simulink model "DP2_Jason_Li"  (R2022a)
settings: Solver=VariableStepAuto  StartTime=0.0  StopTime=100  RelTol=1e-3
model workspace (MATLAB code in the model file):
  | current1=110;
  | current2=110;
  | current3=0;
  | current4=200;
  | const_v=675;
  | 
  | v_set_1=current1*0.3;
  | 
  | v_set_2=current2*0.3;
  | 
  | v_set_3=current3*0.3;
  | 
  | v_set_4=current4*0.3;
  | 
  | P=12;
  | I=1;
  | D=12;
undefined symbols (not defined in the file): D11, Delta, Ion, Lithium
libraries: spsDiodeLib x32, spsSeriesRLCBranchLib x22, spsCurrentMeasurementLib x16, simulink x12, spsMosfetLib x8, slpidlib x8, spsTriangleGeneratorLib x8, spsBatteryLib x4, spsVariableResistorLib x4, spsVoltageMeasurementLib x4, spsThreePhaseTransformerThreeWindingsLib x1, spsThreePhaseVIMeasurementLib x1
(part 2 of 2)

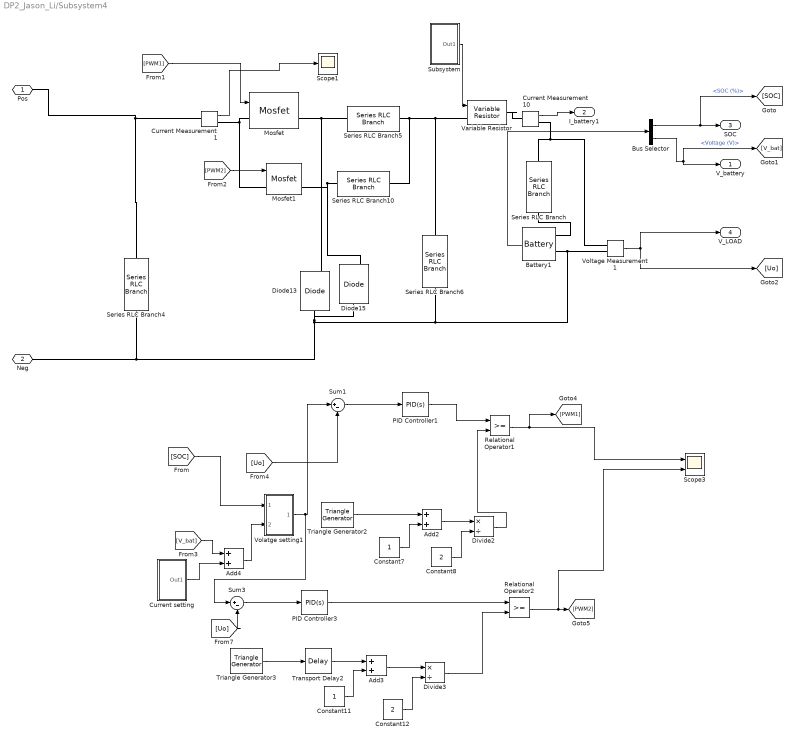
== system DP2_Jason_Li/Subsystem4 ==
  Add2 : Sum
  Add3 : Sum
  Add4 : Sum
  Battery1 : spsBatteryLib/Battery  BatType=Lithium-Ion  ShowTempParam=off  ThermalPreset=no  ShowAgeParam=off  NomV=600  NomQ=150  SOC=0  Batt_Tr=1  PresetModel=off  MaxQ=150  MinV=450  FullV=660  Dis_rate=65.2174  R=1e-7  Normal_OP=135.6522  expZone="[648.2315      7.369565]"  current=[6.5 13 32.5]  Units=Time  Tci=20  NomT=20  T2=-30  MaxQ2=4.8  FullV2=7.1  Normal_OP2=5.655  expZone2="[6.58           1]"  Rca=0.6  ti=2000  Dp=0  Neq0=0  Tsim=1e6  Ta1=25  Qeol=5.4*0.9  Reol=0.013333*1.2  Char_age=[2.3478, 3]  Dis_age=[2.3478, 10]  N1=1500  N2=10500  N3=1000  N4=1400  Ta2=45  N5=950
  Bus Selector : BusSelector  OutputSignals=SOC (%),Voltage (V)
  Constant11 : Constant
  Constant12 : Constant  Value=2
  Constant7 : Constant
  Constant8 : Constant  Value=2
  Current Measurement1 : spsCurrentMeasurementLib/Current Measurement  PhasorSimulation=off  OutputType=Complex  PSBequivalent=0
  Current Measurement10 : spsCurrentMeasurementLib/Current Measurement  PhasorSimulation=off  OutputType=Complex  PSBequivalent=0
  Current setting : Subsystem
  Diode13 : spsDiodeLib/Diode  Ron=0.0001  Lon=0  Vf=0.0001  IC=0  UseSnubber=0  Rs=500  Cs=250e-9  Measurements=on
  Diode15 : spsDiodeLib/Diode  Ron=0.0001  Lon=0  Vf=0.0001  IC=0  UseSnubber=0  Rs=500  Cs=250e-9  Measurements=on
  Divide2 : Product  Inputs=*/
  Divide3 : Product  Inputs=*/
  Mosfet : spsMosfetLib/Mosfet  Ron=0.1  Lon=0  Rd=0.01  Vfd=0  IC=0  Rs=1e5  Cs=inf  Measurements=on
  Mosfet1 : spsMosfetLib/Mosfet  Ron=0.1  Lon=0  Rd=0.01  Vfd=0  IC=0  Rs=1e5  Cs=inf  Measurements=on
  PID Controller1 : slpidlib/PID Controller  Controller=PID  Form=Parallel  TimeDomain=Continuous-time  UseExternalTs=off  SampleTime=-1  IntegratorMethod=Forward Euler  FilterMethod=Forward Euler  ControllerParametersSource=internal  P=P  I=I  UseKiTs=off  D=D  N=100  UseFilter=on  TunerSelectOption=Frequency Response Based  InitialConditionSource=internal  InitialConditionForIntegrator=0  InitialConditionForFilter=0  DifferentiatorICPrevScaledInput=0  ExternalReset=none  TrackingMode=off  Kt=1  LimitOutput=off  SatLimitsSource=internal  UpperSaturationLimit=inf  LowerSaturationLimit=-inf  LinearizeAsGain=on  AntiWindupMode=none  Kb=1  POutMin=[]  POutMax=[]  IOutMin=[]  IOutMax=[]  DOutMin=[]  DOutMax=[]  NOutMin=[]  NOutMax=[]  SumOutMin=[]  SumOutMax=[]  SaturationOutMin=[]  SaturationOutMax=[]  PParamMin=[]  PParamMax=[]  IParamMin=[]  IParamMax=[]  DParamMin=[]  DParamMax=[]  NParamMin=[]  NParamMax=[]  KbParamMin=[]  KbParamMax=[]  KtParamMin=[]  KtParamMax=[]  KbOutMin=[]  KbOutMax=[]  KtOutMin=[]  KtOutMax=[]  IntegratorOutMin=[]  IntegratorOutMax=[]  FilterOutMin=[]  FilterOutMax=[]  SumI1OutMin=[]  SumI1OutMax=[]  SumI2OutMin=[]  SumI2OutMax=[]  SumI3OutMin=[]  SumI3OutMax=[]  SumI4OutMin=[]  SumI4OutMax=[]  SumDOutMin=[]  SumDOutMax=[]  DifferentiatorOutMin=[]  DifferentiatorOutMax=[]  FilterDiffOutCoefMin=[]  FilterDiffOutCoefMax=[]  ReciprocalOutMin=[]  ReciprocalOutMax=[]  SumDenOutMin=[]  SumDenOutMax=[]  SumNumOutMin=[]  SumNumOutMax=[]  DivideOutMin=[]  DivideOutMax=[]  UdiffTsProdOutMin=[]  UdiffTsProdOutMax=[]  NTsProdOutMin=[]  NTsProdOutMax=[]  UintegralTsProdOutMin=[]  UintegralTsProdOutMax=[]  UngainTsProdOutMin=[]  UngainTsProdOutMax=[]  IntegratorContinuousStateAttributes=''  IntegratorStateMustResolveToSignalObject=off  IntegratorRTWStateStorageClass=Auto  FilterContinuousStateAttributes=''  FilterStateMustResolveToSignalObject=off  FilterRTWStateStorageClass=Auto  ParallelPVariant=InternalParameters  IdealPVariant=Disabled  IVariant=InternalParameters  DVariant=InternalParameters  IntegratorVariant=Continuous  SatVariant=Disabled  AWVariant=Passthrough  PCopyVariant=Disabled  TRVariant=Disabled  FdbkBlocksVariant=Forward  IdealPFdbkVariant=Disabled  SatFdbkVariant=Disabled  DerivativeFilterVariant=ContFilter  NVariant=InternalParameters  NCopyVariant=Disabled  FilterICVariant=InternalICsFilter  IntegratorICVariant=InternalICs  ExternalResetVariant=Disabled  TRSumVariant=Passthrough  SumFdbkVariant=Disabled  SumVariant=Sum_PID  TsampFilterVariant=InternalTs  TsampNgainVariant=Passthrough  TsampIntegralVariant=Passthrough  ExternalSaturationOutDataTypeStr=Inherit: Same as second input  aMode=0
  PID Controller3 : slpidlib/PID Controller  Controller=PID  Form=Parallel  TimeDomain=Continuous-time  UseExternalTs=off  SampleTime=-1  IntegratorMethod=Forward Euler  FilterMethod=Forward Euler  ControllerParametersSource=internal  P=P  I=I  UseKiTs=off  D=D  N=100  UseFilter=on  TunerSelectOption=Transfer Function Based (PID Tuner App)  InitialConditionSource=internal  InitialConditionForIntegrator=0  InitialConditionForFilter=0  DifferentiatorICPrevScaledInput=0  ExternalReset=none  TrackingMode=off  Kt=1  LimitOutput=off  SatLimitsSource=internal  UpperSaturationLimit=inf  LowerSaturationLimit=-inf  LinearizeAsGain=on  AntiWindupMode=none  Kb=1  POutMin=[]  POutMax=[]  IOutMin=[]  IOutMax=[]  DOutMin=[]  DOutMax=[]  NOutMin=[]  NOutMax=[]  SumOutMin=[]  SumOutMax=[]  SaturationOutMin=[]  SaturationOutMax=[]  PParamMin=[]  PParamMax=[]  IParamMin=[]  IParamMax=[]  DParamMin=[]  DParamMax=[]  NParamMin=[]  NParamMax=[]  KbParamMin=[]  KbParamMax=[]  KtParamMin=[]  KtParamMax=[]  KbOutMin=[]  KbOutMax=[]  KtOutMin=[]  KtOutMax=[]  IntegratorOutMin=[]  IntegratorOutMax=[]  FilterOutMin=[]  FilterOutMax=[]  SumI1OutMin=[]  SumI1OutMax=[]  SumI2OutMin=[]  SumI2OutMax=[]  SumI3OutMin=[]  SumI3OutMax=[]  SumI4OutMin=[]  SumI4OutMax=[]  SumDOutMin=[]  SumDOutMax=[]  DifferentiatorOutMin=[]  DifferentiatorOutMax=[]  FilterDiffOutCoefMin=[]  FilterDiffOutCoefMax=[]  ReciprocalOutMin=[]  ReciprocalOutMax=[]  SumDenOutMin=[]  SumDenOutMax=[]  SumNumOutMin=[]  SumNumOutMax=[]  DivideOutMin=[]  DivideOutMax=[]  UdiffTsProdOutMin=[]  UdiffTsProdOutMax=[]  NTsProdOutMin=[]  NTsProdOutMax=[]  UintegralTsProdOutMin=[]  UintegralTsProdOutMax=[]  UngainTsProdOutMin=[]  UngainTsProdOutMax=[]  IntegratorContinuousStateAttributes=''  IntegratorStateMustResolveToSignalObject=off  IntegratorRTWStateStorageClass=Auto  FilterContinuousStateAttributes=''  FilterStateMustResolveToSignalObject=off  FilterRTWStateStorageClass=Auto  ParallelPVariant=InternalParameters  IdealPVariant=Disabled  IVariant=InternalParameters  DVariant=InternalParameters  IntegratorVariant=Continuous  SatVariant=Disabled  AWVariant=Passthrough  PCopyVariant=Disabled  TRVariant=Disabled  FdbkBlocksVariant=Forward  IdealPFdbkVariant=Disabled  SatFdbkVariant=Disabled  DerivativeFilterVariant=ContFilter  NVariant=InternalParameters  NCopyVariant=Disabled  FilterICVariant=InternalICsFilter  IntegratorICVariant=InternalICs  ExternalResetVariant=Disabled  TRSumVariant=Passthrough  SumFdbkVariant=Disabled  SumVariant=Sum_PID  TsampFilterVariant=InternalTs  TsampNgainVariant=Passthrough  TsampIntegralVariant=Passthrough  ExternalSaturationOutDataTypeStr=Inherit: Same as second input  aMode=0
  Relational Operator1 : RelationalOperator  OutDataTypeStr=boolean  RndMeth=Simplest  InputSameDT=off
  Relational Operator2 : RelationalOperator  OutDataTypeStr=boolean  RndMeth=Simplest  InputSameDT=off
  Scope1 : Scope
  Scope3 : Scope  NumInputPorts=2
  Series RLC Branch : spsSeriesRLCBranchLib/Series RLC Branch  LConnTagsString=__new0  RConnTagsString=__new0  BranchType=R  Resistance=0.3  Inductance=1e-3  SetiL0=off  InitialCurrent=0  Capacitance=1e-6  Setx0=off  InitialVoltage=0  Measurements=None
  Series RLC Branch10 : spsSeriesRLCBranchLib/Series RLC Branch  LConnTagsString=__new0  RConnTagsString=__new0  BranchType=L  Resistance=0  Inductance=0.5  SetiL0=off  InitialCurrent=0  Capacitance=0.1e-3  Setx0=off  InitialVoltage=0  Measurements=None
  Series RLC Branch4 : spsSeriesRLCBranchLib/Series RLC Branch  LConnTagsString=__new0  RConnTagsString=__new0  BranchType=C  Resistance=0  Inductance=0  SetiL0=off  InitialCurrent=0  Capacitance=1.5e-3  Setx0=off  InitialVoltage=0  Measurements=None
  Series RLC Branch5 : spsSeriesRLCBranchLib/Series RLC Branch  LConnTagsString=__new0  RConnTagsString=__new0  BranchType=L  Resistance=0  Inductance=0.5  SetiL0=off  InitialCurrent=0  Capacitance=0.1e-3  Setx0=off  InitialVoltage=0  Measurements=None
  Series RLC Branch6 : spsSeriesRLCBranchLib/Series RLC Branch  LConnTagsString=__new0  RConnTagsString=__new0  BranchType=C  Resistance=0  Inductance=0  SetiL0=off  InitialCurrent=0  Capacitance=1.5e-3  Setx0=off  InitialVoltage=0  Measurements=None
  Subsystem : Subsystem
  Sum1 : Sum  Inputs=|+-
  Sum3 : Sum  Inputs=|+-
  Transport Delay2 : TransportDelay  DelayTime=0.5/10000
  Triangle Generator2 : spsTriangleGeneratorLib/Triangle Generator  Freq=10e3  Phase=0  Ts=0
  Triangle Generator3 : spsTriangleGeneratorLib/Triangle Generator  Freq=10e3  Phase=0  Ts=0
  Variable Resistor : spsVariableResistorLib/Variable Resistor  Rabsmin=1e-3
      settings: SourceProductBaseCode=PS
  Volatge setting1 : Subsystem
  Voltage Measurement1 : spsVoltageMeasurementLib/Voltage Measurement  PhasorSimulation=off  OutputType=Complex  PSBequivalent=0
  Pos : PMIOPort  Side=Left
  Neg : PMIOPort  Port=2  Side=Left
  V_battery : Outport
  I_battery1 : Outport  Port=2
  SOC : Outport  Port=3
  V_LOAD : Outport  Port=4
  wires:
  [PWM1] -> Mosfet/1
  [PWM2] -> Mosfet1/1
  Current Measurement1/1 -> Scope1/1
  Constant12/1 -> Divide3/2
  [Uo] -> Sum1/2
  Triangle Generator2/1 -> Add2/1
  Constant8/1 -> Divide2/2
  Bus Selector/2 -> [V_bat], V_battery/1  "<Voltage (V)>"
  Divide3/1 -> Relational Operator2/2
  Current setting/1(Out1) -> Add4/2
  Divide2/1 -> Relational Operator1/2
  Transport Delay2/1 -> Add3/1
  Add2/1 -> Divide2/1
  Relational Operator1/1 -> Scope3/1, [PWM1]
  PID Controller3/1 -> Relational Operator2/1
  Battery1/1 -> Bus Selector/1
  Triangle Generator3/1 -> Transport Delay2/1
  [Uo] -> Sum3/2
  PID Controller1/1 -> Relational Operator1/1
  Add3/1 -> Divide3/1
  Current Measurement10/1 -> I_battery1/1
  Relational Operator2/1 -> Scope3/2, [PWM2]
  Sum3/1 -> PID Controller3/1
  Constant11/1 -> Add3/2
  Voltage Measurement1/1 -> V_LOAD/1, [Uo]
  Constant7/1 -> Add2/2
  Sum1/1 -> PID Controller1/1
  Bus Selector/1 -> [SOC], SOC/1  "<SOC (%)>"
  Subsystem/1(Out1) -> Variable Resistor/1
  Add4/1 -> Volatge setting1/2(const_I)
  Volatge setting1/1(Out1) -> Sum3/1, Sum1/1
  [SOC] -> Volatge setting1/1(SOC)
  [V_bat] -> Add4/1
  connections:
  Mosfet1/LConn1 -- Current Measurement1/RConn1 -- Mosfet/LConn1
  Variable Resistor/LConn1 -- Series RLC Branch5/RConn1 -- Series RLC Branch10/RConn1 -- Series RLC Branch6/LConn1
  Series RLC Branch10/LConn1 -- Mosfet1/RConn1 -- Diode15/RConn1
  Mosfet/RConn1 -- Series RLC Branch5/LConn1 -- Diode13/RConn1
  Series RLC Branch4/LConn1 -- Pos/RConn1 -- Current Measurement1/LConn1
  Diode15/LConn1 -- Diode13/LConn1 -- Battery1/LConn2 -- Voltage Measurement1/LConn2 -- Series RLC Branch6/RConn1 -- Neg/RConn1 -- Series RLC Branch4/RConn1
  Current Measurement10/RConn1 -- Voltage Measurement1/LConn1 -- Series RLC Branch/LConn1
  Battery1/LConn1 -- Series RLC Branch/RConn1
  Variable Resistor/RConn1 -- Current Measurement10/LConn1

== system DP2_Jason_Li/Subsystem1/Current setting ==
  Constant9 : Constant  Value=v_set_1
  Ramp1 : simulink/Sources/Ramp  slope=5  start=0  InitialOutput=0
  Switch : Switch  Criteria=u2 > Threshold  Threshold=v_set_1  SaturateOnIntegerOverflow=off  InputSameDT=off
  Out1 : Outport
  wires:
  Ramp1/1 -> Switch/3, Switch/2
  Switch/1 -> Out1/1
  Constant9/1 -> Switch/1

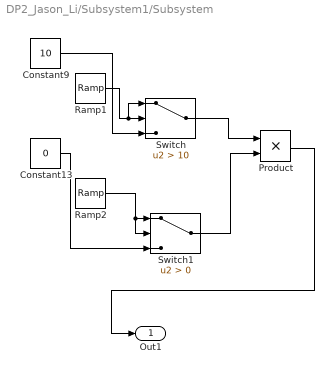
== system DP2_Jason_Li/Subsystem1/Subsystem ==
  Constant13 : Constant  Value=0
  Constant9 : Constant  Value=10
  Product : Product
  Ramp1 : simulink/Sources/Ramp  slope=-10  start=0  InitialOutput=100
  Ramp2 : simulink/Sources/Ramp  slope=-0.4  start=0  InitialOutput=1.9
  Switch : Switch  Criteria=u2 > Threshold  Threshold=10  SaturateOnIntegerOverflow=off  InputSameDT=off
  Switch1 : Switch  Criteria=u2 > Threshold  SaturateOnIntegerOverflow=off  InputSameDT=off
  Out1 : Outport
  wires:
  Constant9/1 -> Switch/3
  Ramp1/1 -> Switch/1, Switch/2
  Product/1 -> Out1/1
  Constant13/1 -> Switch1/3
  Switch/1 -> Product/1
  Switch1/1 -> Product/2
  Ramp2/1 -> Switch1/2, Switch1/1

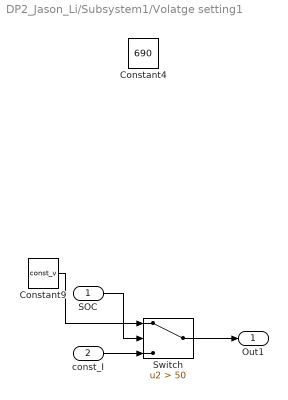
== system DP2_Jason_Li/Subsystem1/Volatge setting1 ==
  SOC : Inport
  const_I : Inport  Port=2
  Constant4 : Constant  Value=690
  Constant9 : Constant  Value=const_v
  Switch : Switch  Criteria=u2 > Threshold  Threshold=50  SaturateOnIntegerOverflow=off  InputSameDT=off
  Out1 : Outport
  wires:
  SOC/1 -> Switch/2
  Switch/1 -> Out1/1
  Constant9/1 -> Switch/1
  const_I/1 -> Switch/3

== system DP2_Jason_Li/Subsystem2/Current setting ==
  Constant9 : Constant  Value=v_set_2
  Ramp1 : simulink/Sources/Ramp  slope=5  start=0  InitialOutput=0
  Switch : Switch  Criteria=u2 > Threshold  Threshold=v_set_1  SaturateOnIntegerOverflow=off  InputSameDT=off
  Out1 : Outport
  wires:
  Ramp1/1 -> Switch/3, Switch/2
  Switch/1 -> Out1/1
  Constant9/1 -> Switch/1

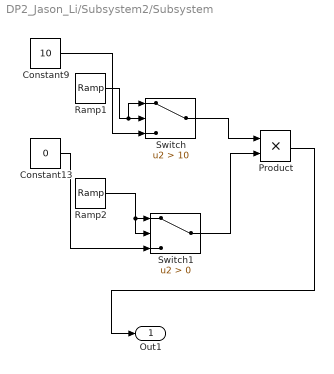
== system DP2_Jason_Li/Subsystem2/Subsystem ==
  Constant13 : Constant  Value=0
  Constant9 : Constant  Value=10
  Product : Product
  Ramp1 : simulink/Sources/Ramp  slope=-10  start=0  InitialOutput=100
  Ramp2 : simulink/Sources/Ramp  slope=-0.4  start=0  InitialOutput=1.9
  Switch : Switch  Criteria=u2 > Threshold  Threshold=10  SaturateOnIntegerOverflow=off  InputSameDT=off
  Switch1 : Switch  Criteria=u2 > Threshold  SaturateOnIntegerOverflow=off  InputSameDT=off
  Out1 : Outport
  wires:
  Constant9/1 -> Switch/3
  Ramp1/1 -> Switch/1, Switch/2
  Product/1 -> Out1/1
  Constant13/1 -> Switch1/3
  Switch/1 -> Product/1
  Switch1/1 -> Product/2
  Ramp2/1 -> Switch1/2, Switch1/1

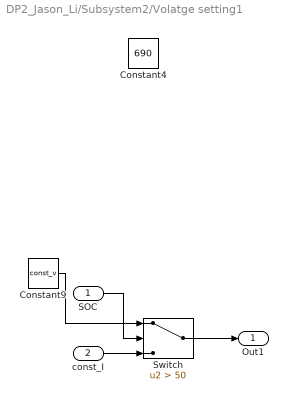
== system DP2_Jason_Li/Subsystem2/Volatge setting1 ==
  SOC : Inport
  const_I : Inport  Port=2
  Constant4 : Constant  Value=690
  Constant9 : Constant  Value=const_v
  Switch : Switch  Criteria=u2 > Threshold  Threshold=50  SaturateOnIntegerOverflow=off  InputSameDT=off
  Out1 : Outport
  wires:
  SOC/1 -> Switch/2
  Switch/1 -> Out1/1
  Constant9/1 -> Switch/1
  const_I/1 -> Switch/3

== system DP2_Jason_Li/Subsystem3/Current setting ==
  Constant9 : Constant  Value=v_set_3
  Ramp1 : simulink/Sources/Ramp  slope=5  start=0  InitialOutput=0
  Switch : Switch  Criteria=u2 > Threshold  Threshold=v_set_1  SaturateOnIntegerOverflow=off  InputSameDT=off
  Out1 : Outport
  wires:
  Ramp1/1 -> Switch/3, Switch/2
  Switch/1 -> Out1/1
  Constant9/1 -> Switch/1

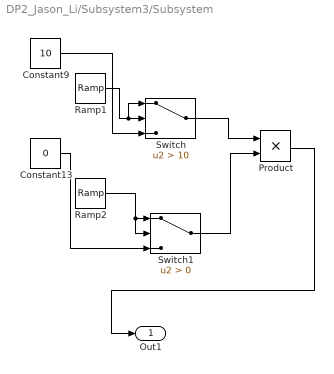
== system DP2_Jason_Li/Subsystem3/Subsystem ==
  Constant13 : Constant  Value=0
  Constant9 : Constant  Value=10
  Product : Product
  Ramp1 : simulink/Sources/Ramp  slope=-10  start=0  InitialOutput=100
  Ramp2 : simulink/Sources/Ramp  slope=-0.4  start=0  InitialOutput=1.9
  Switch : Switch  Criteria=u2 > Threshold  Threshold=10  SaturateOnIntegerOverflow=off  InputSameDT=off
  Switch1 : Switch  Criteria=u2 > Threshold  SaturateOnIntegerOverflow=off  InputSameDT=off
  Out1 : Outport
  wires:
  Constant9/1 -> Switch/3
  Ramp1/1 -> Switch/1, Switch/2
  Product/1 -> Out1/1
  Constant13/1 -> Switch1/3
  Switch/1 -> Product/1
  Switch1/1 -> Product/2
  Ramp2/1 -> Switch1/2, Switch1/1

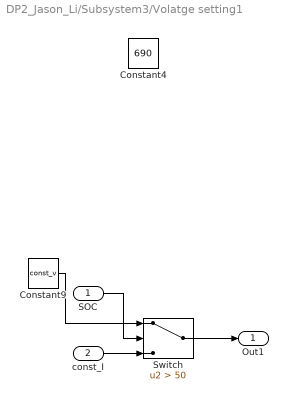
== system DP2_Jason_Li/Subsystem3/Volatge setting1 ==
  SOC : Inport
  const_I : Inport  Port=2
  Constant4 : Constant  Value=690
  Constant9 : Constant  Value=const_v
  Switch : Switch  Criteria=u2 > Threshold  Threshold=50  SaturateOnIntegerOverflow=off  InputSameDT=off
  Out1 : Outport
  wires:
  SOC/1 -> Switch/2
  Switch/1 -> Out1/1
  Constant9/1 -> Switch/1
  const_I/1 -> Switch/3

== system DP2_Jason_Li/Subsystem4/Current setting ==
  Constant9 : Constant  Value=v_set_4
  Ramp1 : simulink/Sources/Ramp  slope=5  start=0  InitialOutput=0
  Switch : Switch  Criteria=u2 > Threshold  Threshold=v_set_1  SaturateOnIntegerOverflow=off  InputSameDT=off
  Out1 : Outport
  wires:
  Ramp1/1 -> Switch/3, Switch/2
  Switch/1 -> Out1/1
  Constant9/1 -> Switch/1

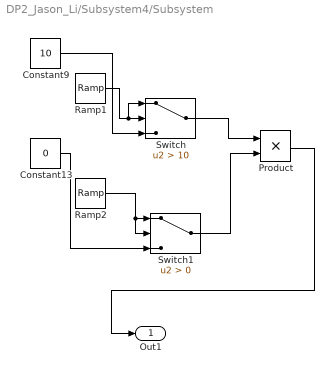
== system DP2_Jason_Li/Subsystem4/Subsystem ==
  Constant13 : Constant  Value=0
  Constant9 : Constant  Value=10
  Product : Product
  Ramp1 : simulink/Sources/Ramp  slope=-10  start=0  InitialOutput=100
  Ramp2 : simulink/Sources/Ramp  slope=-0.4  start=0  InitialOutput=1.9
  Switch : Switch  Criteria=u2 > Threshold  Threshold=10  SaturateOnIntegerOverflow=off  InputSameDT=off
  Switch1 : Switch  Criteria=u2 > Threshold  SaturateOnIntegerOverflow=off  InputSameDT=off
  Out1 : Outport
  wires:
  Constant9/1 -> Switch/3
  Ramp1/1 -> Switch/1, Switch/2
  Product/1 -> Out1/1
  Constant13/1 -> Switch1/3
  Switch/1 -> Product/1
  Switch1/1 -> Product/2
  Ramp2/1 -> Switch1/2, Switch1/1

== system DP2_Jason_Li/Subsystem4/Volatge setting1 ==
  SOC : Inport
  const_I : Inport  Port=2
  Constant4 : Constant  Value=690
  Constant9 : Constant  Value=const_v
  Switch : Switch  Criteria=u2 > Threshold  Threshold=50  SaturateOnIntegerOverflow=off  InputSameDT=off
  Out1 : Outport
  wires:
  SOC/1 -> Switch/2
  Switch/1 -> Out1/1
  Constant9/1 -> Switch/1
  const_I/1 -> Switch/3
